simulink model "autopilota_v_15_last"  (R2020b)
settings: Solver=ode4  StartTime=0.0  StopTime=300  FixedStep=0.02  RelTol=1e-3
values from neighbouring files (symbols this model uses):
  attuatore_Amax = 20*(pi/180)    (= 0.349065850399)    [v2021_10_27_avvioSITL.m]    (also in v2021_10_27_calcoloAerodinamica.m)
  attuatore_Amin = -20*(pi/180)    (= -0.349065850399)    [v2021_10_27_avvioSITL.m]
  attuatore_Emax = 25*(pi/180)    (= 0.436332312999)    [v2021_10_27_avvioSITL.m]    (also in v2021_10_27_calcoloAerodinamica.m)
  attuatore_Emin = -25*(pi/180)    (= -0.436332312999)    [v2021_10_27_avvioSITL.m]
  attuatore_Rmax = 25*(pi/180)    (= 0.436332312999)    [v2021_10_27_avvioSITL.m]    (also in v2021_10_27_calcoloAerodinamica.m)
  attuatore_Rmin = -25*(pi/180)    (= -0.436332312999)    [v2021_10_27_avvioSITL.m]
  attuatore_Tmax = 0.99    [v2021_10_27_avvioSITL.m]
  attuatore_Tmin = 0    [v2021_10_27_avvioSITL.m]
  bias = [baccxINI,baccyINI,bacczINI,bpINI,bqINI,brINI]    [v2021_10_27_avvioSITL.m]
  final_h = 35    [v2021_10_27_avvioSITL.m]
  interventoA_05 = 20*0.8    (= 16)    [v2021_10_27_avvioSITL.m]
  interventoA_1 = 10    [v2021_10_27_avvioSITL.m]
  interventoE_05 = 25*0.8    (= 20)    [v2021_10_27_avvioSITL.m]
  interventoE_1 = 10    [v2021_10_27_avvioSITL.m]
  interventoT = 1*0.6    (= 0.6)    [v2021_10_27_avvioSITL.m]
  inv_A = 1    [v2021_10_27_avvioSITL.m]
  inv_comp_h = 1    [v2021_10_27_avvioSITL.m]
  inv_E = 1    [v2021_10_27_avvioSITL.m]
  inv_R = 1    [v2021_10_27_avvioSITL.m]
  inv_T = 1    [v2021_10_27_avvioSITL.m]
  K_AW_B_AP_quota = 1000    [v2021_10_27_avvioSITL.m]
  K_AW_B_becc = -250    [v2021_10_27_avvioSITL.m]
  K_AW_B_imb = 0    [v2021_10_27_avvioSITL.m]
  K_AW_B_roll = 500    [v2021_10_27_avvioSITL.m]
  K_imb_inv = -0.001306    [v2021_10_27_avvioSITL.m]
  Kd_AP_rotta = 0.995    [v2021_10_27_avvioSITL.m]
  Kd_h_app = 0.085    [v2021_10_27_avvioSITL.m]
  Kd_h_flare = 0.01    [v2021_10_27_avvioSITL.m]
  Ki_AP_quota_select = 0.01936    [v2021_10_27_avvioSITL.m]
  Ki_AP_rotta = 0.002    [v2021_10_27_avvioSITL.m]
  Ki_AP_vel = 0.025175    [v2021_10_27_avvioSITL.m]
  Ki_becch = -0.1963    [v2021_10_27_avvioSITL.m]
  Ki_h_app = 0.055    [v2021_10_27_avvioSITL.m]
  Ki_h_cruise = 0.008    [v2021_10_27_avvioSITL.m]
  Ki_h_flare = 0.07    [v2021_10_27_avvioSITL.m]
  Ki_roll = 0.004528    [v2021_10_27_avvioSITL.m]
  Kp_AP_quota_hold_h = 0.5503    [v2021_10_27_avvioSITL.m]
  Kp_AP_quota_hold_l = 0.5503    [v2021_10_27_avvioSITL.m]
  Kp_AP_quota_select = 0.02647    [v2021_10_27_avvioSITL.m]
  Kp_AP_rotta = 0.520    (= 0.52)    [v2021_10_27_avvioSITL.m]
  Kp_AP_vel = 0.132175    [v2021_10_27_avvioSITL.m]
  Kp_becch = -0.30    (= -0.3)    [v2021_10_27_avvioSITL.m]
  Kp_comp_h = 0.035    [v2021_10_27_avvioSITL.m]
  Kp_h_app_max = 0.086    [v2021_10_27_avvioSITL.m]
  Kp_h_app_min = 0.01    [v2021_10_27_avvioSITL.m]
  Kp_h_cruise = 0.04    [v2021_10_27_avvioSITL.m]
  Kp_h_flare = 0.1    [v2021_10_27_avvioSITL.m]
  Kp_imb = 0.0019415    [v2021_10_27_avvioSITL.m]
  Kp_p = 0.006913    [v2021_10_27_avvioSITL.m]
  Kp_q = -0.025    [v2021_10_27_avvioSITL.m]
  Kp_roll = 0.0718    [v2021_10_27_avvioSITL.m]
  Kp_Rotta_ATO = 4    [v2021_10_27_avvioSITL.m]
  Kp_Rotta_psi = -0.01    [v2021_10_27_avvioSITL.m]
  Q1B = [    2e-15;     2e-15 ... (first row only)    [COV_F1B.m]
  R1B = [     2e-14;             2e-14 ... (first row only)    [COV_F1B.m]
  safe_phi = 55    [v2021_10_27_avvioSITL.m]
  safe_V = 40    [v2021_10_27_avvioSITL.m]
  Sensor_Offsets = [0,0,0]    [v2021_10_27_avvioSITL.m]
  T_cal = 0.4    [v2021_10_27_avvioSITL.m]
  theta_rot = 10    [v2021_10_27_avvioSITL.m]
  time_alarm_SAFE = 300    [v2021_10_27_avvioSITL.m]
  tsamp = 0.02    [v2021_10_27_avvioSITL.m]
  update = [2,2,2]    [v2021_10_27_avvioSITL.m]
  V_max = 35    [v2021_10_27_avvioSITL.m]
  V_stall = 15    [v2021_10_27_avvioSITL.m]
  vd_ini = 0    [v2021_10_27_avvioSITL.m]
  vel_wp1_al = 25    [v2021_10_27_avvioSITL.m]
  vel_wp2_al = 20    [v2021_10_27_avvioSITL.m]
undefined symbols (not defined in the file or in its folder): DiscIntNeverNeededParam, Newton, Raphson, t_AP
libraries: simulink_extras x41, pid_lib x8, dspsigops x4, simulink x3, aerolibtransform2sys x2, aerolibtransform2 x2, cstblocks x1, aerosimlib x1
(part 7 of 11)

== matlab function autopilota_v_15_last/MISURE DA SENSORI FILTRATE/Filtro di Kalman/MATLAB Function1 ==
  settings: updateMethod=DISCRETE  sampleTime=0.02
  data: Lat_K output; z1 input; z2 input; z3 input; z4 input; z5 input; z6 input; z7 input; z8 input; z9 input; z10 input; z11 input; z12 input; z13 input; z14 input; z15 input; clock_GPS input; clock_MTi input; Long_K output; h_K output; v_K output; vd_K output; phi_K output; theta_K output; psi_K output; p_K output; q_K output; r_K output; errore_5 output; errore_9 output; imbardata output
function [Lat_K,Long_K,h_K,v_K,vd_K,phi_K,theta_K,psi_K,p_K,q_K,r_K,errore_5,errore_9,imbardata] = kalmanfilter(z1, z2, z3, z4, z5, z6, z7, z8, z9, z10, z11, z12, z13, z14, z15, clock_GPS, clock_MTi)
%#codegen                                                  
%     x_prd = [latitudine_Ini;...        % lat        
%              longitudine_Ini;...       % long
%              quota_Ini;...             % quota
%              velnord_Ini;...           % vel. nord
%              velest_Ini;...            % vel. est
%              veldown_Ini;...           % vel. salita/discesa
%              rollio_Ini;...            % rollio
%              beccheggio_Ini;...        % beccheggio
%              imbardata_Ini;...         % imbardata
%              accnord_Ini;...           % acc nord
%              accest_Ini;...            % acc est
%              accdown_Ini;...           % acc down
%              velrollio_Ini;...         % vel. rollio
%              velbeccheggio_Ini;...     % vel. beccheggio
%              velimbardata_Ini;...      % vel. imbardata
%              biasaccx_Ini;...          % bias accx 
%              biasaccy_Ini;...          % bias accy
%              biasaccz_Ini;...          % bias accz
%              biasvelrollio_Ini;...     % bias vel. angolare rollio
%              biasvelbeccheggio_Ini;... % bias vel. angolare beccheggio
%              biasvelimbardata_Ini];    % bias vel algolare imbardata

persistent x_prd
persistent p_prd 

a = 6378137; % earth radius (m)

g=9.81;      % gravity constant

Z = [z1;z2;z3;z4;z5;z6;z7;z8;z9;z10;z11;z12;z13;z14;z15];

infinito = 1e40;

dt=0.02;




%%%%%%%%%%%%%%%%%%%%%%%%%%%%%%%%%%%%%%%%%%%%%%
%% Initial (predicted) state and covariance %%
%%%%%%%%%%%%%%%%%%%%%%%%%%%%%%%%%%%%%%%%%%%%%%

% Condizioni iniziali filtro di Kalman

% latitudineINI = 0.73117;
% 
% longitudineINI = 0.21803;
% 
% quotaINI = 100;
% 
% velnordINI = 25;
% 
% velestINI = -0.05;
% 
% veldownINI = 0;
% 
% phiINI = 0;
% 
% thetaINI = -0.01;
% 
% psiINI = 0;
% 
% accnordINI = 0;
% 
% accestINI = 0;
% 
% accdownINI = 0;
% 
% pINI = 0;
% 
% qINI = 0;
% 
% rINI = 0;
% 
% biasaccxINI = 0.02;
% 
% biasaccyINI = 0.02;
% 
% biasacczINI = 0.02;
% 
% biaspINI = 9.7e-5;
% 
% biasqINI = 9.7e-5;
% 
% biasrINI = 9.7e-5;

latitudineINI = 41.7831770578592199*pi/180;   

longitudineINI = 12.2399282455444336*pi/180;

quotaINI =5;

velnordINI = 25;

velestINI = 0;

veldownINI = 0;

vINI = 0;

phiINI = 0;

thetaINI = -0.01;

psiINI = 0;

accnordINI = 0;

accestINI = 0;

accdownINI = 0;

pINI = 0;

qINI = 0;

rINI = 0;

biasaccxINI = 0.02;

biasaccyINI = 0.02;

biasacczINI = 0.02;

biaspINI = 9.7e-5;

biasqINI = 9.7e-5;

biasrINI = 9.7e-5;



% Inizializzo stato e covarianza

if isempty(x_prd)
   
    x_prd =[ latitudineINI;...
             longitudineINI;...
             quotaINI;...
             velnordINI;...
             velestINI;...
             veldownINI;...
             phiINI;...
             thetaINI;...
             psiINI;...
             accnordINI;...
             accestINI;...
             accdownINI;...
             pINI;...
             qINI;...
             rINI;...
             biasaccxINI;...
             biasaccyINI;...
             biasacczINI;...
             biaspINI;...
             biasqINI;...
             biasrINI;];

 	p_prd = zeros(21,21);
end

%%%%%%%%%%%%%%%%%%%%%%%%%%%%%
%%      Sensor Offsets     %%
%%%%%%%%%%%%%%%%%%%%%%%%%%%%%

rxIMU = 0.15;

ryIMU = 0;

rzIMU = 0;

rxGPS = -0.1;

ryGPS = 0;

rzGPS = -0.1;


%%%%%%%%%%%%%%%%%%%%%%%%%%%%%%
%% Process noise covariance %%
%%%%%%%%%%%%%%%%%%%%%%%%%%%%%%

Q = [ 3e-11;...%Lat
      4e-11;...%Long
      3e-5;...%h
      8.5e-9;...%vn
      9.5e-8;...%ve
      4e-8;...%vd
      1e-7;...%phi
      1e-7;...%theta
      5e-6;...%psi
      30;...%an
      30;...%ae
      1e-2;...%ad
      4e-06;...%p
      4e-06;...%q
      5e-06;...%r
      6e-15;...%baccx
      6e-15;...%baccy
      6e-15;...%baccz
      6e-15;...%bp
      6e-15;...%bq
      6e-15];  %br
  
%%%%%%%%%%%%%%%%%%%%%%%%%%%
%% Predicted measurement %%  
%%%%%%%%%%%%%%%%%%%%%%%%%%%
    
Y_prd =[x_prd(1);
        x_prd(2);
        x_prd(3);  %(SensorePressione)
        (abs(x_prd(5) - (cos(x_prd(9))*sin(x_prd(7)) - cos(x_prd(7))*sin(x_prd(9))*sin(x_prd(8)))*(x_prd(13)*ryGPS - x_prd(14)*rxGPS) - (cos(x_prd(7))*cos(x_prd(9)) + sin(x_prd(7))*sin(x_prd(9))*sin(x_prd(8)))*(x_prd(13)*rzGPS - x_prd(15)*rxGPS) + cos(x_prd(8))*sin(x_prd(9))*(x_prd(14)*rzGPS - x_prd(15)*ryGPS))^2 + abs(x_prd(4) + (sin(x_prd(7))*sin(x_prd(9)) + cos(x_prd(7))*cos(x_prd(9))*sin(x_prd(8)))*(x_prd(13)*ryGPS - x_prd(14)*rxGPS) + (cos(x_prd(7))*sin(x_prd(9)) - cos(x_prd(9))*sin(x_prd(7))*sin(x_prd(8)))*(x_prd(13)*rzGPS - x_prd(15)*rxGPS) + cos(x_prd(9))*cos(x_prd(8))*(x_prd(14)*rzGPS - x_prd(15)*ryGPS))^2)^(1/2);
        atan2(x_prd(5),x_prd(4));
        x_prd(6) - sin(x_prd(8))*(x_prd(14)*rzGPS - x_prd(15)*ryGPS) - cos(x_prd(8))*sin(x_prd(7))*(x_prd(13)*rzGPS - x_prd(15)*rxGPS) + cos(x_prd(7))*cos(x_prd(8))*(x_prd(13)*ryGPS - x_prd(14)*rxGPS);
        x_prd(7);
        x_prd(8);
        x_prd(9);
        x_prd(13)+x_prd(19);
        x_prd(14)+x_prd(20);
        x_prd(15)+x_prd(21);
        cos(x_prd(8))*cos(x_prd(9))*x_prd(10) + cos(x_prd(8))*sin(x_prd(9))*x_prd(11) - sin(x_prd(8))*(x_prd(12)-g) + x_prd(14)*(x_prd(13)*ryIMU - x_prd(14)*rxIMU) + x_prd(15)*(x_prd(13)*rzIMU - x_prd(15)*rxIMU) + x_prd(16);
        ( sin(x_prd(7))*sin(x_prd(8))*cos(x_prd(9)) - cos(x_prd(7))*sin(x_prd(9)) )*x_prd(10) + ( sin(x_prd(7))*sin(x_prd(8))*sin(x_prd(9)) + cos(x_prd(7))*cos(x_prd(9)) )*x_prd(11) + sin(x_prd(7))*cos(x_prd(8))*(x_prd(12)-g) - x_prd(13)*(x_prd(13)*ryIMU - x_prd(14)*rxIMU) + x_prd(15)*(x_prd(14)*rzIMU - x_prd(15)*ryIMU) + x_prd(17);
        ( cos(x_prd(7))*sin(x_prd(8))*cos(x_prd(9)) + sin(x_prd(7))*sin(x_prd(9)) )*x_prd(10) + ( cos(x_prd(7))*sin(x_prd(8))*sin(x_prd(9)) - sin(x_prd(7))*cos(x_prd(9)) )*x_prd(11) + cos(x_prd(7))*cos(x_prd(8))*(x_prd(12)-g) - x_prd(13)*(x_prd(13)*rzIMU - x_prd(15)*rxIMU) - x_prd(14)*(x_prd(14)*rzIMU - x_prd(15)*ryIMU) + x_prd(18)];
		
%%%%%%%%%%%%%%%%%%%%%%%%%%%
%% Linearize measurement %%
%%%%%%%%%%%%%%%%%%%%%%%%%%%

vn = x_prd(4); ve = x_prd(5);  phi  = x_prd(7); theta = x_prd(8); psi = x_prd(9);

an  = x_prd(10); ae = x_prd(11); ad = x_prd(12); p = x_prd(13); q = x_prd(14); r = x_prd(15); 

H = [ 1, 0, 0,                                                                                                                                                                                                                                                                                                                                                                                                                                                                                                                                                                                                                                                                                                                                                                                                                                0,                                                                                                                                                                                                                                                                                                                                                                                                                                                                                                                                                                                                                                                                                                                                                                                                                                0, 0,                                                                                                                                                                                                                                                                                                                                                                                                                                                                                                                                                                                                                                                                                                                                                                                                                                                                                                                                                                                                                                                                                                                                                                                                                                                                                                                                                                                                                                                                                                                                                       0,                                                                                                                                                                                                                                                                                                                                                                                                                                                                                                                                                                                                                                                                                                                                                                                                                                                                                                                                                                                                                                                                                                                                                                                                                                                                                                                                                                                                                                                                                                                                                    0,                                                                                                                                                                                                                                                                                                                                                                                                                                                                                                                                                                                                                                                                                                                                                                                                                                                                                                                                                                                                                                                                                                                                                                                                                                                                                                                                                                                                                                                                                                                                                                                                                                           0,                                                0,                                                0,                   0,                                                                                                                                                                                                                                                                                                                                                                                                                                                                                                                                                                                                                                                                                                                                                                                                                                                                                                                                                                                                                                                                                                                                                                                                                                                                                                                                                                                                                                                                                               0,                                                                                                                                                                                                                                                                                                                                                                                                                                                                                                                                                                                                                                                                                                                                                                                                                                                                                                                                                                                                                                                                                                                                                                                                                                                                                                                                                                                                                                  0,                                                                                                                                                                                                                                                                                                                                                                                                                                                                                                                                                                                                                                                                                                                                                                                                                                                                                                                                                                                                                                                                                                                                                                                                                                                                                                                                                                                                                                  0, 0, 0, 0, 0, 0, 0;...
      0, 1, 0,                                                                                                                                                                                                                                                                                                                                                                                                                                                                                                                                                                                                                                                                                                                                                                                                                                0,                                                                                                                                                                                                                                                                                                                                                                                                                                                                                                                                                                                                                                                                                                                                                                                                                                0, 0,                                                                                                                                                                                                                                                                                                                                                                                                                                                                                                                                                                                                                                                                                                                                                                                                                                                                                                                                                                                                                                                                                                                                                                                                                                                                                                                                                                                                                                                                                                                                                       0,                                                                                                                                                                                                                                                                                                                                                                                                                                                                                                                                                                                                                                                                                                                                                                                                                                                                                                                                                                                                                                                                                                                                                                                                                                                                                                                                                                                                                                                                                                                                                    0,                                                                                                                                                                                                                                                                                                                                                                                                                                                                                                                                                                                                                                                                                                                                                                                                                                                                                                                                                                                                                                                                                                                                                                                                                                                                                                                                                                                                                                                                                                                                                                                                                                           0,                                                0,                                                0,                   0,                                                                                                                                                                                                                                                                                                                                                                                                                                                                                                                                                                                                                                                                                                                                                                                                                                                                                                                                                                                                                                                                                                                                                                                                                                                                                                                                                                                                                                                                                               0,                                                                                                                                                                                                                                                                                                                                                                                                                                                                                                                                                                                                                                                                                                                                                                                                                                                                                                                                                                                                                                                                                                                                                                                                                                                                                                                                                                                                                                  0,                                                                                                                                                                                                                                                                                                                                                                                                                                                                                                                                                                                                                                                                                                                                                                                                                                                                                                                                                                                                                                                                                                                                                                                                                                                                                                                                                                                                                                  0, 0, 0, 0, 0, 0, 0;...
      0, 0, 1,                                                                                                                                                                                                                                                                                                                                                                                                                                                                                                                                                                                                                                                                                                                                                                                                                                0,                                                                                                                                                                                                                                                                                                                                                                                                                                                                                                                                                                                                                                                                                                                                                                                                                                0, 0,                                                                                                                                                                                                                                                                                                                                                                                                                                                                                                                                                                                                                                                                                                                                                                                                                                                                                                                                                                                                                                                                                                                                                                                                                                                                                                                                                                                                                                                                                                                                                       0,                                                                                                                                                                                                                                                                                                                                                                                                                                                                                                                                                                                                                                                                                                                                                                                                                                                                                                                                                                                                                                                                                                                                                                                                                                                                                                                                                                                                                                                                                                                                                    0,                                                                                                                                                                                                                                                                                                                                                                                                                                                                                                                                                                                                                                                                                                                                                                                                                                                                                                                                                                                                                                                                                                                                                                                                                                                                                                                                                                                                                                                                                                                                                                                                                                           0,                                                0,                                                0,                   0,                                                                                                                                                                                                                                                                                                                                                                                                                                                                                                                                                                                                                                                                                                                                                                                                                                                                                                                                                                                                                                                                                                                                                                                                                                                                                                                                                                                                                                                                                               0,                                                                                                                                                                                                                                                                                                                                                                                                                                                                                                                                                                                                                                                                                                                                                                                                                                                                                                                                                                                                                                                                                                                                                                                                                                                                                                                                                                                                                                  0,                                                                                                                                                                                                                                                                                                                                                                                                                                                                                                                                                                                                                                                                                                                                                                                                                                                                                                                                                                                                                                                                                                                                                                                                                                                                                                                                                                                                                                  0, 0, 0, 0, 0, 0, 0;...
      0, 0, 0, (abs(vn + (sin(phi)*sin(psi) + cos(phi)*cos(psi)*sin(theta))*(p*ryGPS - q*rxGPS) + (cos(phi)*sin(psi) - cos(psi)*sin(phi)*sin(theta))*(p*rzGPS - r*rxGPS) + cos(psi)*cos(theta)*(q*rzGPS - r*ryGPS))*sign(vn + (sin(phi)*sin(psi) + cos(phi)*cos(psi)*sin(theta))*(p*ryGPS - q*rxGPS) + (cos(phi)*sin(psi) - cos(psi)*sin(phi)*sin(theta))*(p*rzGPS - r*rxGPS) + cos(psi)*cos(theta)*(q*rzGPS - r*ryGPS)))/(abs(vn + (sin(phi)*sin(psi) + cos(phi)*cos(psi)*sin(theta))*(p*ryGPS - q*rxGPS) + (cos(phi)*sin(psi) - cos(psi)*sin(phi)*sin(theta))*(p*rzGPS - r*rxGPS) + cos(psi)*cos(theta)*(q*rzGPS - r*ryGPS))^2 + abs(ve - (cos(psi)*sin(phi) - cos(phi)*sin(psi)*sin(theta))*(p*ryGPS - q*rxGPS) - (cos(phi)*cos(psi) + sin(phi)*sin(psi)*sin(theta))*(p*rzGPS - r*rxGPS) + cos(theta)*sin(psi)*(q*rzGPS - r*ryGPS))^2)^(1/2), (abs(ve - (cos(psi)*sin(phi) - cos(phi)*sin(psi)*sin(theta))*(p*ryGPS - q*rxGPS) - (cos(phi)*cos(psi) + sin(phi)*sin(psi)*sin(theta))*(p*rzGPS - r*rxGPS) + cos(theta)*sin(psi)*(q*rzGPS - r*ryGPS))*sign(ve - (cos(psi)*sin(phi) - cos(phi)*sin(psi)*sin(theta))*(p*ryGPS - q*rxGPS) - (cos(phi)*cos(psi) + sin(phi)*sin(psi)*sin(theta))*(p*rzGPS - r*rxGPS) + cos(theta)*sin(psi)*(q*rzGPS - r*ryGPS)))/(abs(vn + (sin(phi)*sin(psi) + cos(phi)*cos(psi)*sin(theta))*(p*ryGPS - q*rxGPS) + (cos(phi)*sin(psi) - cos(psi)*sin(phi)*sin(theta))*(p*rzGPS - r*rxGPS) + cos(psi)*cos(theta)*(q*rzGPS - r*ryGPS))^2 + abs(ve - (cos(psi)*sin(phi) - cos(phi)*sin(psi)*sin(theta))*(p*ryGPS - q*rxGPS) - (cos(phi)*cos(psi) + sin(phi)*sin(psi)*sin(theta))*(p*rzGPS - r*rxGPS) + cos(theta)*sin(psi)*(q*rzGPS - r*ryGPS))^2)^(1/2), 0, (2*abs(vn + (sin(phi)*sin(psi) + cos(phi)*cos(psi)*sin(theta))*(p*ryGPS - q*rxGPS) + (cos(phi)*sin(psi) - cos(psi)*sin(phi)*sin(theta))*(p*rzGPS - r*rxGPS) + cos(psi)*cos(theta)*(q*rzGPS - r*ryGPS))*sign(vn + (sin(phi)*sin(psi) + cos(phi)*cos(psi)*sin(theta))*(p*ryGPS - q*rxGPS) + (cos(phi)*sin(psi) - cos(psi)*sin(phi)*sin(theta))*(p*rzGPS - r*rxGPS) + cos(psi)*cos(theta)*(q*rzGPS - r*ryGPS))*((cos(phi)*sin(psi) - cos(psi)*sin(phi)*sin(theta))*(p*ryGPS - q*rxGPS) - (sin(phi)*sin(psi) + cos(phi)*cos(psi)*sin(theta))*(p*rzGPS - r*rxGPS)) - 2*abs(ve - (cos(psi)*sin(phi) - cos(phi)*sin(psi)*sin(theta))*(p*ryGPS - q*rxGPS) - (cos(phi)*cos(psi) + sin(phi)*sin(psi)*sin(theta))*(p*rzGPS - r*rxGPS) + cos(theta)*sin(psi)*(q*rzGPS - r*ryGPS))*sign(ve - (cos(psi)*sin(phi) - cos(phi)*sin(psi)*sin(theta))*(p*ryGPS - q*rxGPS) - (cos(phi)*cos(psi) + sin(phi)*sin(psi)*sin(theta))*(p*rzGPS - r*rxGPS) + cos(theta)*sin(psi)*(q*rzGPS - r*ryGPS))*((cos(phi)*cos(psi) + sin(phi)*sin(psi)*sin(theta))*(p*ryGPS - q*rxGPS) - (cos(psi)*sin(phi) - cos(phi)*sin(psi)*sin(theta))*(p*rzGPS - r*rxGPS)))/(2*(abs(vn + (sin(phi)*sin(psi) + cos(phi)*cos(psi)*sin(theta))*(p*ryGPS - q*rxGPS) + (cos(phi)*sin(psi) - cos(psi)*sin(phi)*sin(theta))*(p*rzGPS - r*rxGPS) + cos(psi)*cos(theta)*(q*rzGPS - r*ryGPS))^2 + abs(ve - (cos(psi)*sin(phi) - cos(phi)*sin(psi)*sin(theta))*(p*ryGPS - q*rxGPS) - (cos(phi)*cos(psi) + sin(phi)*sin(psi)*sin(theta))*(p*rzGPS - r*rxGPS) + cos(theta)*sin(psi)*(q*rzGPS - r*ryGPS))^2)^(1/2)), -(2*abs(vn + (sin(phi)*sin(psi) + cos(phi)*cos(psi)*sin(theta))*(p*ryGPS - q*rxGPS) + (cos(phi)*sin(psi) - cos(psi)*sin(phi)*sin(theta))*(p*rzGPS - r*rxGPS) + cos(psi)*cos(theta)*(q*rzGPS - r*ryGPS))*sign(vn + (sin(phi)*sin(psi) + cos(phi)*cos(psi)*sin(theta))*(p*ryGPS - q*rxGPS) + (cos(phi)*sin(psi) - cos(psi)*sin(phi)*sin(theta))*(p*rzGPS - r*rxGPS) + cos(psi)*cos(theta)*(q*rzGPS - r*ryGPS))*(cos(psi)*sin(theta)*(q*rzGPS - r*ryGPS) - cos(phi)*cos(psi)*cos(theta)*(p*ryGPS - q*rxGPS) + cos(psi)*cos(theta)*sin(phi)*(p*rzGPS - r*rxGPS)) + 2*abs(ve - (cos(psi)*sin(phi) - cos(phi)*sin(psi)*sin(theta))*(p*ryGPS - q*rxGPS) - (cos(phi)*cos(psi) + sin(phi)*sin(psi)*sin(theta))*(p*rzGPS - r*rxGPS) + cos(theta)*sin(psi)*(q*rzGPS - r*ryGPS))*sign(ve - (cos(psi)*sin(phi) - cos(phi)*sin(psi)*sin(theta))*(p*ryGPS - q*rxGPS) - (cos(phi)*cos(psi) + sin(phi)*sin(psi)*sin(theta))*(p*rzGPS - r*rxGPS) + cos(theta)*sin(psi)*(q*rzGPS - r*ryGPS))*(sin(psi)*sin(theta)*(q*rzGPS - r*ryGPS) - cos(phi)*cos(theta)*sin(psi)*(p*ryGPS - q*rxGPS) + cos(theta)*sin(phi)*sin(psi)*(p*rzGPS - r*rxGPS)))/(2*(abs(vn + (sin(phi)*sin(psi) + cos(phi)*cos(psi)*sin(theta))*(p*ryGPS - q*rxGPS) + (cos(phi)*sin(psi) - cos(psi)*sin(phi)*sin(theta))*(p*rzGPS - r*rxGPS) + cos(psi)*cos(theta)*(q*rzGPS - r*ryGPS))^2 + abs(ve - (cos(psi)*sin(phi) - cos(phi)*sin(psi)*sin(theta))*(p*ryGPS - q*rxGPS) - (cos(phi)*cos(psi) + sin(phi)*sin(psi)*sin(theta))*(p*rzGPS - r*rxGPS) + cos(theta)*sin(psi)*(q*rzGPS - r*ryGPS))^2)^(1/2)), (2*abs(vn + (sin(phi)*sin(psi) + cos(phi)*cos(psi)*sin(theta))*(p*ryGPS - q*rxGPS) + (cos(phi)*sin(psi) - cos(psi)*sin(phi)*sin(theta))*(p*rzGPS - r*rxGPS) + cos(psi)*cos(theta)*(q*rzGPS - r*ryGPS))*sign(vn + (sin(phi)*sin(psi) + cos(phi)*cos(psi)*sin(theta))*(p*ryGPS - q*rxGPS) + (cos(phi)*sin(psi) - cos(psi)*sin(phi)*sin(theta))*(p*rzGPS - r*rxGPS) + cos(psi)*cos(theta)*(q*rzGPS - r*ryGPS))*((cos(psi)*sin(phi) - cos(phi)*sin(psi)*sin(theta))*(p*ryGPS - q*rxGPS) + (cos(phi)*cos(psi) + sin(phi)*sin(psi)*sin(theta))*(p*rzGPS - r*rxGPS) - cos(theta)*sin(psi)*(q*rzGPS - r*ryGPS)) + 2*abs(ve - (cos(psi)*sin(phi) - cos(phi)*sin(psi)*sin(theta))*(p*ryGPS - q*rxGPS) - (cos(phi)*cos(psi) + sin(phi)*sin(psi)*sin(theta))*(p*rzGPS - r*rxGPS) + cos(theta)*sin(psi)*(q*rzGPS - r*ryGPS))*sign(ve - (cos(psi)*sin(phi) - cos(phi)*sin(psi)*sin(theta))*(p*ryGPS - q*rxGPS) - (cos(phi)*cos(psi) + sin(phi)*sin(psi)*sin(theta))*(p*rzGPS - r*rxGPS) + cos(theta)*sin(psi)*(q*rzGPS - r*ryGPS))*((sin(phi)*sin(psi) + cos(phi)*cos(psi)*sin(theta))*(p*ryGPS - q*rxGPS) + (cos(phi)*sin(psi) - cos(psi)*sin(phi)*sin(theta))*(p*rzGPS - r*rxGPS) + cos(psi)*cos(theta)*(q*rzGPS - r*ryGPS)))/(2*(abs(vn + (sin(phi)*sin(psi) + cos(phi)*cos(psi)*sin(theta))*(p*ryGPS - q*rxGPS) + (cos(phi)*sin(psi) - cos(psi)*sin(phi)*sin(theta))*(p*rzGPS - r*rxGPS) + cos(psi)*cos(theta)*(q*rzGPS - r*ryGPS))^2 + abs(ve - (cos(psi)*sin(phi) - cos(phi)*sin(psi)*sin(theta))*(p*ryGPS - q*rxGPS) - (cos(phi)*cos(psi) + sin(phi)*sin(psi)*sin(theta))*(p*rzGPS - r*rxGPS) + cos(theta)*sin(psi)*(q*rzGPS - r*ryGPS))^2)^(1/2)),                                                0,                                                0,                   0, (2*abs(vn + (sin(phi)*sin(psi) + cos(phi)*cos(psi)*sin(theta))*(p*ryGPS - q*rxGPS) + (cos(phi)*sin(psi) - cos(psi)*sin(phi)*sin(theta))*(p*rzGPS - r*rxGPS) + cos(psi)*cos(theta)*(q*rzGPS - r*ryGPS))*sign(vn + (sin(phi)*sin(psi) + cos(phi)*cos(psi)*sin(theta))*(p*ryGPS - q*rxGPS) + (cos(phi)*sin(psi) - cos(psi)*sin(phi)*sin(theta))*(p*rzGPS - r*rxGPS) + cos(psi)*cos(theta)*(q*rzGPS - r*ryGPS))*(ryGPS*(sin(phi)*sin(psi) + cos(phi)*cos(psi)*sin(theta)) + rzGPS*(cos(phi)*sin(psi) - cos(psi)*sin(phi)*sin(theta))) - 2*abs(ve - (cos(psi)*sin(phi) - cos(phi)*sin(psi)*sin(theta))*(p*ryGPS - q*rxGPS) - (cos(phi)*cos(psi) + sin(phi)*sin(psi)*sin(theta))*(p*rzGPS - r*rxGPS) + cos(theta)*sin(psi)*(q*rzGPS - r*ryGPS))*sign(ve - (cos(psi)*sin(phi) - cos(phi)*sin(psi)*sin(theta))*(p*ryGPS - q*rxGPS) - (cos(phi)*cos(psi) + sin(phi)*sin(psi)*sin(theta))*(p*rzGPS - r*rxGPS) + cos(theta)*sin(psi)*(q*rzGPS - r*ryGPS))*(ryGPS*(cos(psi)*sin(phi) - cos(phi)*sin(psi)*sin(theta)) + rzGPS*(cos(phi)*cos(psi) + sin(phi)*sin(psi)*sin(theta))))/(2*(abs(vn + (sin(phi)*sin(psi) + cos(phi)*cos(psi)*sin(theta))*(p*ryGPS - q*rxGPS) + (cos(phi)*sin(psi) - cos(psi)*sin(phi)*sin(theta))*(p*rzGPS - r*rxGPS) + cos(psi)*cos(theta)*(q*rzGPS - r*ryGPS))^2 + abs(ve - (cos(psi)*sin(phi) - cos(phi)*sin(psi)*sin(theta))*(p*ryGPS - q*rxGPS) - (cos(phi)*cos(psi) + sin(phi)*sin(psi)*sin(theta))*(p*rzGPS - r*rxGPS) + cos(theta)*sin(psi)*(q*rzGPS - r*ryGPS))^2)^(1/2)), -(2*abs(vn + (sin(phi)*sin(psi) + cos(phi)*cos(psi)*sin(theta))*(p*ryGPS - q*rxGPS) + (cos(phi)*sin(psi) - cos(psi)*sin(phi)*sin(theta))*(p*rzGPS - r*rxGPS) + cos(psi)*cos(theta)*(q*rzGPS - r*ryGPS))*sign(vn + (sin(phi)*sin(psi) + cos(phi)*cos(psi)*sin(theta))*(p*ryGPS - q*rxGPS) + (cos(phi)*sin(psi) - cos(psi)*sin(phi)*sin(theta))*(p*rzGPS - r*rxGPS) + cos(psi)*cos(theta)*(q*rzGPS - r*ryGPS))*(rxGPS*(sin(phi)*sin(psi) + cos(phi)*cos(psi)*sin(theta)) - rzGPS*cos(psi)*cos(theta)) - 2*abs(ve - (cos(psi)*sin(phi) - cos(phi)*sin(psi)*sin(theta))*(p*ryGPS - q*rxGPS) - (cos(phi)*cos(psi) + sin(phi)*sin(psi)*sin(theta))*(p*rzGPS - r*rxGPS) + cos(theta)*sin(psi)*(q*rzGPS - r*ryGPS))*sign(ve - (cos(psi)*sin(phi) - cos(phi)*sin(psi)*sin(theta))*(p*ryGPS - q*rxGPS) - (cos(phi)*cos(psi) + sin(phi)*sin(psi)*sin(theta))*(p*rzGPS - r*rxGPS) + cos(theta)*sin(psi)*(q*rzGPS - r*ryGPS))*(rxGPS*(cos(psi)*sin(phi) - cos(phi)*sin(psi)*sin(theta)) + rzGPS*cos(theta)*sin(psi)))/(2*(abs(vn + (sin(phi)*sin(psi) + cos(phi)*cos(psi)*sin(theta))*(p*ryGPS - q*rxGPS) + (cos(phi)*sin(psi) - cos(psi)*sin(phi)*sin(theta))*(p*rzGPS - r*rxGPS) + cos(psi)*cos(theta)*(q*rzGPS - r*ryGPS))^2 + abs(ve - (cos(psi)*sin(phi) - cos(phi)*sin(psi)*sin(theta))*(p*ryGPS - q*rxGPS) - (cos(phi)*cos(psi) + sin(phi)*sin(psi)*sin(theta))*(p*rzGPS - r*rxGPS) + cos(theta)*sin(psi)*(q*rzGPS - r*ryGPS))^2)^(1/2)), -(2*abs(vn + (sin(phi)*sin(psi) + cos(phi)*cos(psi)*sin(theta))*(p*ryGPS - q*rxGPS) + (cos(phi)*sin(psi) - cos(psi)*sin(phi)*sin(theta))*(p*rzGPS - r*rxGPS) + cos(psi)*cos(theta)*(q*rzGPS - r*ryGPS))*sign(vn + (sin(phi)*sin(psi) + cos(phi)*cos(psi)*sin(theta))*(p*ryGPS - q*rxGPS) + (cos(phi)*sin(psi) - cos(psi)*sin(phi)*sin(theta))*(p*rzGPS - r*rxGPS) + cos(psi)*cos(theta)*(q*rzGPS - r*ryGPS))*(rxGPS*(cos(phi)*sin(psi) - cos(psi)*sin(phi)*sin(theta)) + ryGPS*cos(psi)*cos(theta)) - 2*abs(ve - (cos(psi)*sin(phi) - cos(phi)*sin(psi)*sin(theta))*(p*ryGPS - q*rxGPS) - (cos(phi)*cos(psi) + sin(phi)*sin(psi)*sin(theta))*(p*rzGPS - r*rxGPS) + cos(theta)*sin(psi)*(q*rzGPS - r*ryGPS))*sign(ve - (cos(psi)*sin(phi) - cos(phi)*sin(psi)*sin(theta))*(p*ryGPS - q*rxGPS) - (cos(phi)*cos(psi) + sin(phi)*sin(psi)*sin(theta))*(p*rzGPS - r*rxGPS) + cos(theta)*sin(psi)*(q*rzGPS - r*ryGPS))*(rxGPS*(cos(phi)*cos(psi) + sin(phi)*sin(psi)*sin(theta)) - ryGPS*cos(theta)*sin(psi)))/(2*(abs(vn + (sin(phi)*sin(psi) + cos(phi)*cos(psi)*sin(theta))*(p*ryGPS - q*rxGPS) + (cos(phi)*sin(psi) - cos(psi)*sin(phi)*sin(theta))*(p*rzGPS - r*rxGPS) + cos(psi)*cos(theta)*(q*rzGPS - r*ryGPS))^2 + abs(ve - (cos(psi)*sin(phi) - cos(phi)*sin(psi)*sin(theta))*(p*ryGPS - q*rxGPS) - (cos(phi)*cos(psi) + sin(phi)*sin(psi)*sin(theta))*(p*rzGPS - r*rxGPS) + cos(theta)*sin(psi)*(q*rzGPS - r*ryGPS))^2)^(1/2)), 0, 0, 0, 0, 0, 0;...
      0, 0, 0,                                                                                                                                                                                                                                                                                                                                                                                                                                                                                                                                                                                                                                                                                                                                                                                                                -ve/(ve^2 + vn^2),                                                                                                                                                                                                                                                                                                                                                                                                                                                                                                                                                                                                                                                                                                                                                                                                                 vn/(ve^2 + vn^2), 0,                                                                                                                                                                                                                                                                                                                                                                                                                                                                                                                                                                                                                                                                                                                                                                                                                                                                                                                                                                                                                                                                                                                                                                                                                                                                                                                                                                                                                                                                                                                                                       0,                                                                                                                                                                                                                                                                                                                                                                                                                                                                                                                                                                                                                                                                                                                                                                                                                                                                                                                                                                                                                                                                                                                                                                                                                                                                                                                                                                                                                                                                                                                                                    0,                                                                                                                                                                                                                                                                                                                                                                                                                                                                                                                                                                                                                                                                                                                                                                                                                                                                                                                                                                                                                                                                                                                                                                                                                                                                                                                                                                                                                                                                                                                                                                                                                                           0,                                                0,                                                0,                   0,                                                                                                                                                                                                                                                                                                                                                                                                                                                                                                                                                                                                                                                                                                                                                                                                                                                                                                                                                                                                                                                                                                                                                                                                                                                                                                                                                                                                                                                                                               0,                                                                                                                                                                                                                                                                                                                                                                                                                                                                                                                                                                                                                                                                                                                                                                                                                                                                                                                                                                                                                                                                                                                                                                                                                                                                                                                                                                                                                                  0,                                                                                                                                                                                                                                                                                                                                                                                                                                                                                                                                                                                                                                                                                                                                                                                                                                                                                                                                                                                                                                                                                                                                                                                                                                                                                                                                                                                                                                  0, 0, 0, 0, 0, 0, 0;...
      0, 0, 0,                                                                                                                                                                                                                                                                                                                                                                                                                                                                                                                                                                                                                                                                                                                                                                                                                                0,                                                                                                                                                                                                                                                                                                                                                                                                                                                                                                                                                                                                                                                                                                                                                                                                                                0, 1,                                                                                                                                                                                                                                                                                                                                                                                                                                                                                                                                                                                                                                                                                                                                                                                                                                                                                                                                                                                                                                                                                                                                                                                                                                                                                                                                                                                                                                                                     - cos(phi)*cos(theta)*(p*rzGPS - r*rxGPS) - cos(theta)*sin(phi)*(p*ryGPS - q*rxGPS),                                                                                                                                                                                                                                                                                                                                                                                                                                                                                                                                                                                                                                                                                                                                                                                                                                                                                                                                                                                                                                                                                                                                                                                                                                                                                                                                                                                                                                   sin(phi)*sin(theta)*(p*rzGPS - r*rxGPS) - cos(theta)*(q*rzGPS - r*ryGPS) - cos(phi)*sin(theta)*(p*ryGPS - q*rxGPS),                                                                                                                                                                                                                                                                                                                                                                                                                                                                                                                                                                                                                                                                                                                                                                                                                                                                                                                                                                                                                                                                                                                                                                                                                                                                                                                                                                                                                                                                                                                                                                                                                                           0,                                                0,                                                0,                   0,                                                                                                                                                                                                                                                                                                                                                                                                                                                                                                                                                                                                                                                                                                                                                                                                                                                                                                                                                                                                                                                                                                                                                                                                                                                                                                                                                                                                                                           ryGPS*cos(phi)*cos(theta) - rzGPS*cos(theta)*sin(phi),                                                                                                                                                                                                                                                                                                                                                                                                                                                                                                                                                                                                                                                                                                                                                                                                                                                                                                                                                                                                                                                                                                                                                                                                                                                                                                                                                                                     - rzGPS*sin(theta) - rxGPS*cos(phi)*cos(theta),                                                                                                                                                                                                                                                                                                                                                                                                                                                                                                                                                                                                                                                                                                                                                                                                                                                                                                                                                                                                                                                                                                                                                                                                                                                                                                                                                                                       ryGPS*sin(theta) + rxGPS*cos(theta)*sin(phi), 0, 0, 0, 0, 0, 0;...
      0, 0, 0,                                                                                                                                                                                                                                                                                                                                                                                                                                                                                                                                                                                                                                                                                                                                                                                                                                0,                                                                                                                                                                                                                                                                                                                                                                                                                                                                                                                                                                                                                                                                                                                                                                                                                                0, 0,                                                                                                                                                                                                                                                                                                                                                                                                                                                                                                                                                                                                                                                                                                                                                                                                                                                                                                                                                                                                                                                                                                                                                                                                                                                                                                                                                                                                                                                                                                                                                       1,                                                                                                                                                                                                                                                                                                                                                                                                                                                                                                                                                                                                                                                                                                                                                                                                                                                                                                                                                                                                                                                                                                                                                                                                                                                                                                                                                                                                                                                                                                                                                    0,                                                                                                                                                                                                                                                                                                                                                                                                                                                                                                                                                                                                                                                                                                                                                                                                                                                                                                                                                                                                                                                                                                                                                                                                                                                                                                                                                                                                                                                                                                                                                                                                                                           0,                                                0,                                                0,                   0,                                                                                                                                                                                                                                                                                                                                                                                                                                                                                                                                                                                                                                                                                                                                                                                                                                                                                                                                                                                                                                                                                                                                                                                                                                                                                                                                                                                                                                                                                               0,                                                                                                                                                                                                                                                                                                                                                                                                                                                                                                                                                                                                                                                                                                                                                                                                                                                                                                                                                                                                                                                                                                                                                                                                                                                                                                                                                                                                                                  0,                                                                                                                                                                                                                                                                                                                                                                                                                                                                                                                                                                                                                                                                                                                                                                                                                                                                                                                                                                                                                                                                                                                                                                                                                                                                                                                                                                                                                                  0, 0, 0, 0, 0, 0, 0;...
      0, 0, 0,                                                                                                                                                                                                                                                                                                                                                                                                                                                                                                                                                                                                                                                                                                                                                                                                                                0,                                                                                                                                                                                                                                                                                                                                                                                                                                                                                                                                                                                                                                                                                                                                                                                                                                0, 0,                                                                                                                                                                                                                                                                                                                                                                                                                                                                                                                                                                                                                                                                                                                                                                                                                                                                                                                                                                                                                                                                                                                                                                                                                                                                                                                                                                                                                                                                                                                                                       0,                                                                                                                                                                                                                                                                                                                                                                                                                                                                                                                                                                                                                                                                                                                                                                                                                                                                                                                                                                                                                                                                                                                                                                                                                                                                                                                                                                                                                                                                                                                                                    1,                                                                                                                                                                                                                                                                                                                                                                                                                                                                                                                                                                                                                                                                                                                                                                                                                                                                                                                                                                                                                                                                                                                                                                                                                                                                                                                                                                                                                                                                                                                                                                                                                                           0,                                                0,                                                0,                   0,                                                                                                                                                                                                                                                                                                                                                                                                                                                                                                                                                                                                                                                                                                                                                                                                                                                                                                                                                                                                                                                                                                                                                                                                                                                                                                                                                                                                                                                                                               0,                                                                                                                                                                                                                                                                                                                                                                                                                                                                                                                                                                                                                                                                                                                                                                                                                                                                                                                                                                                                                                                                                                                                                                                                                                                                                                                                                                                                                                  0,                                                                                                                                                                                                                                                                                                                                                                                                                                                                                                                                                                                                                                                                                                                                                                                                                                                                                                                                                                                                                                                                                                                                                                                                                                                                                                                                                                                                                                  0, 0, 0, 0, 0, 0, 0;...
      0, 0, 0,                                                                                                                                                                                                                                                                                                                                                                                                                                                                                                                                                                                                                                                                                                                                                                                                                                0,                                                                                                                                                                                                                                                                                                                                                                                                                                                                                                                                                                                                                                                                                                                                                                                                                                0, 0,                                                                                                                                                                                                                                                                                                                                                                                                                                                                                                                                                                                                                                                                                                                                                                                                                                                                                                                                                                                                                                                                                                                                                                                                                                                                                                                                                                                                                                                                                                                                                       0,                                                                                                                                                                                                                                                                                                                                                                                                                                                                                                                                                                                                                                                                                                                                                                                                                                                                                                                                                                                                                                                                                                                                                                                                                                                                                                                                                                                                                                                                                                                                                    0,                                                                                                                                                                                                                                                                                                                                                                                                                                                                                                                                                                                                                                                                                                                                                                                                                                                                                                                                                                                                                                                                                                                                                                                                                                                                                                                                                                                                                                                                                                                                                                                                                                           1,                                                0,                                                0,                   0,                                                                                                                                                                                                                                                                                                                                                                                                                                                                                                                                                                                                                                                                                                                                                                                                                                                                                                                                                                                                                                                                                                                                                                                                                                                                                                                                                                                                                                                                                               0,                                                                                                                                                                                                                                                                                                                                                                                                                                                                                                                                                                                                                                                                                                                                                                                                                                                                                                                                                                                                                                                                                                                                                                                                                                                                                                                                                                                                                                  0,                                                                                                                                                                                                                                                                                                                                                                                                                                                                                                                                                                                                                                                                                                                                                                                                                                                                                                                                                                                                                                                                                                                                                                                                                                                                                                                                                                                                                                  0, 0, 0, 0, 0, 0, 0;...
      0, 0, 0,                                                                                                                                                                                                                                                                                                                                                                                                                                                                                                                                                                                                                                                                                                                                                                                                                                0,                                                                                                                                                                                                                                                                                                                                                                                                                                                                                                                                                                                                                                                                                                                                                                                                                                0, 0,                                                                                                                                                                                                                                                                                                                                                                                                                                                                                                                                                                                                                                                                                                                                                                                                                                                                                                                                                                                                                                                                                                                                                                                                                                                                                                                                                                                                                                                                                                                                                       0,                                                                                                                                                                                                                                                                                                                                                                                                                                                                                                                                                                                                                                                                                                                                                                                                                                                                                                                                                                                                                                                                                                                                                                                                                                                                                                                                                                                                                                                                                                                                                    0,                                                                                                                                                                                                                                                                                                                                                                                                                                                                                                                                                                                                                                                                                                                                                                                                                                                                                                                                                                                                                                                                                                                                                                                                                                                                                                                                                                                                                                                                                                                                                                                                                                           0,                                                0,                                                0,                   0,                                                                                                                                                                                                                                                                                                                                                                                                                                                                                                                                                                                                                                                                                                                                                                                                                                                                                                                                                                                                                                                                                                                                                                                                                                                                                                                                                                                                                                                                                               1,                                                                                                                                                                                                                                                                                                                                                                                                                                                                                                                                                                                                                                                                                                                                                                                                                                                                                                                                                                                                                                                                                                                                                                                                                                                                                                                                                                                                                                  0,                                                                                                                                                                                                                                                                                                                                                                                                                                                                                                                                                                                                                                                                                                                                                                                                                                                                                                                                                                                                                                                                                                                                                                                                                                                                                                                                                                                                                                  0, 0, 0, 0, 1, 0, 0;...
      0, 0, 0,                                                                                                                                                                                                                                                                                                                                                                                                                                                                                                                                                                                                                                                                                                                                                                                                                                0,                                                                                                                                                                                                                                                                                                                                                                                                                                                                                                                                                                                                                                                                                                                                                                                                                                0, 0,                                                                                                                                                                                                                                                                                                                                                                                                                                                                                                                                                                                                                                                                                                                                                                                                                                                                                                                                                                                                                                                                                                                                                                                                                                                                                                                                                                                                                                                                                                                                                       0,                                                                                                                                                                                                                                                                                                                                                                                                                                                                                                                                                                                                                                                                                                                                                                                                                                                                                                                                                                                                                                                                                                                                                                                                                                                                                                                                                                                                                                                                                                                                                    0,                                                                                                                                                                                                                                                                                                                                                                                                                                                                                                                                                                                                                                                                                                                                                                                                                                                                                                                                                                                                                                                                                                                                                                                                                                                                                                                                                                                                                                                                                                                                                                                                                                           0,                                                0,                                                0,                   0,                                                                                                                                                                                                                                                                                                                                                                                                                                                                                                                                                                                                                                                                                                                                                                                                                                                                                                                                                                                                                                                                                                                                                                                                                                                                                                                                                                                                                                                                                               0,                                                                                                                                                                                                                                                                                                                                                                                                                                                                                                                                                                                                                                                                                                                                                                                                                                                                                                                                                                                                                                                                                                                                                                                                                                                                                                                                                                                                                                  1,                                                                                                                                                                                                                                                                                                                                                                                                                                                                                                                                                                                                                                                                                                                                                                                                                                                                                                                                                                                                                                                                                                                                                                                                                                                                                                                                                                                                                                  0, 0, 0, 0, 0, 1, 0;...
      0, 0, 0,                                                                                                                                                                                                                                                                                                                                                                                                                                                                                                                                                                                                                                                                                                                                                                                                                                0,                                                                                                                                                                                                                                                                                                                                                                                                                                                                                                                                                                                                                                                                                                                                                                                                                                0, 0,                                                                                                                                                                                                                                                                                                                                                                                                                                                                                                                                                                                                                                                                                                                                                                                                                                                                                                                                                                                                                                                                                                                                                                                                                                                                                                                                                                                                                                                                                                                                                       0,                                                                                                                                                                                                                                                                                                                                                                                                                                                                                                                                                                                                                                                                                                                                                                                                                                                                                                                                                                                                                                                                                                                                                                                                                                                                                                                                                                                                                                                                                                                                                    0,                                                                                                                                                                                                                                                                                                                                                                                                                                                                                                                                                                                                                                                                                                                                                                                                                                                                                                                                                                                                                                                                                                                                                                                                                                                                                                                                                                                                                                                                                                                                                                                                                                           0,                                                0,                                                0,                   0,                                                                                                                                                                                                                                                                                                                                                                                                                                                                                                                                                                                                                                                                                                                                                                                                                                                                                                                                                                                                                                                                                                                                                                                                                                                                                                                                                                                                                                                                                               0,                                                                                                                                                                                                                                                                                                                                                                                                                                                                                                                                                                                                                                                                                                                                                                                                                                                                                                                                                                                                                                                                                                                                                                                                                                                                                                                                                                                                                                  0,                                                                                                                                                                                                                                                                                                                                                                                                                                                                                                                                                                                                                                                                                                                                                                                                                                                                                                                                                                                                                                                                                                                                                                                                                                                                                                                                                                                                                                  1, 0, 0, 0, 0, 0, 1;...
